simulink model "AccTarSel_PLAN_CTRL"  (R2018b)
settings: Solver=FixedStepDiscrete  StartTime=0.0  StopTime=inf  FixedStep=0.01  RelTol=1e-3
PostLoadFcn:
  | if any(exist('dsrtsu_mdlpostloadfcn', 'file') ~= 0), dsrtsu_mdlpostloadfcn('Execute', bdroot); end
undefined symbols (not defined in the file or in its folder): P_CutInEnable, P_dObjDrvOffMax, P_dObjDrvOffMin, P_dvarYMax4PO, P_dyCutInThres, P_kapHystThres, P_PlausIntegDisable, P_plausMin4PO, P_probExistMin4PO, P_StandObjEnable, P_tAxTrackNegLower, P_tAxTrackNegUpper, P_tAxTrackPosLower, P_tAxTrackPosUpper, P_tCurvFilt, P_tCutInFilt, P_tFiltAxAbsPONegFast, P_tFiltAxAbsPONegSlow, P_tFiltAxAbsPOPosFast, P_tFiltAxAbsPOPosSlow, P_tFiltAxAbsPOStand, P_tFiltVxAxPOFast, P_tFiltVxAxPOSlow, P_tMinDrvPhase, P_vObjDrvOff, P_vStandStill, P_vStandStillHyst, P_vyCutInThres
libraries: LPFilter x6, simulink x3
(part 1 of 3)
settings Model: DSRTSU_INTERNAL_RTI_VER=540  DSRTSU_INTERNAL_RTI_TYPE=rti1401  RTICANMMDATA=struct('GeneralSetupData',struct('modelroot','E:\jiangyunchengGit\laneChangeFunctional\ACC','generalsettings',struct('filesettings',struct('destfolder',struct('Name','RTICANMM_FILES','Check',1),'buildfolder',struct('Name','.','Check',1),'AbsDestfolder',struct('Name','E:\jiangyunchengGit\laneChangeFunctional\ACC\RTICANMM_FILES'),'AbsBuildfolder',struct('Name','E:\jiangyunchengGit\laneChangeFunctional\ACC'))),'options',struct('addpaths',1,'rmpaths',1,'addtrcexclusion',logical(1),'cannavigator',struct('checkmonitoring',0),'show_usrtrc',0,'use_usrtrc',0),'advanced',struct('options',ones(1,100)),'MPSetup',{{}},'RTI',struct('Type','RTI1401','Ver','7.12','Date','02-May-2019'),'modelname','AccTarSel_PLAN_CTRL','block','AccTarSel_PLAN_CTRL'))  DSRTSU_INTERNAL_RTIFPGA=130  Creator=linqi  LastModifiedBy=lenovo
settings OptimizationCC: BlockReduction=off  ConditionallyExecuteInputs=off  OptimizeBlockIOStorage=off  BufferReuse=off  GlobalBufferReuse=off  ExpressionFolding=off  PassReuseOutputArgsThreshold=0  LocalBlockOutputs=off  OptimizeDataStoreBuffers=off  BusAssignmentInplaceUpdate=off  OptimizationLevel=level0
settings DebuggingCC: ParameterTunabilityLossMsg=error
settings HardwareCC: ProdBitPerPointer=32  ProdBitPerSizeT=32  ProdBitPerPtrDiffT=32  ProdLargestAtomicInteger=Integer  ProdEndianess=BigEndian  ProdWordSize=32  ProdHWDeviceType=Custom Processor->Custom  TargetIntDivRoundTo=Zero  TargetEndianess=BigEndian  TargetHWDeviceType=Custom Processor->Custom
settings ModelReferenceCC: ModelReferenceNumInstancesAllowed=Single
settings SFSimCC: MATLABDynamicMemAlloc=off
settings RTWCC: SystemTargetFile=rti1401.tlc  MakeCommand=make_rti  TemplateMakefile=rti1401.tmf  Description=dSPACE DS1401 Hardware Platform  GenerateReport=on  LaunchReport=on
settings CodeAppCC: OperatorAnnotations=on
settings STFCustomTargetCC: ParMdlRefBuildCompliant=on  SystemTargetFile=rti1401.tlc
settings GRTTargetCC: TargetLangStandard=C89/C90 (ANSI)  CompOptLevelCompliant=off  ConcurrentExecutionCompliant=off  CombineOutputUpdateFcns=off  MatFileLogging=off  CPPClassGenCompliant=off  UseToolchainInfoCompliant=off

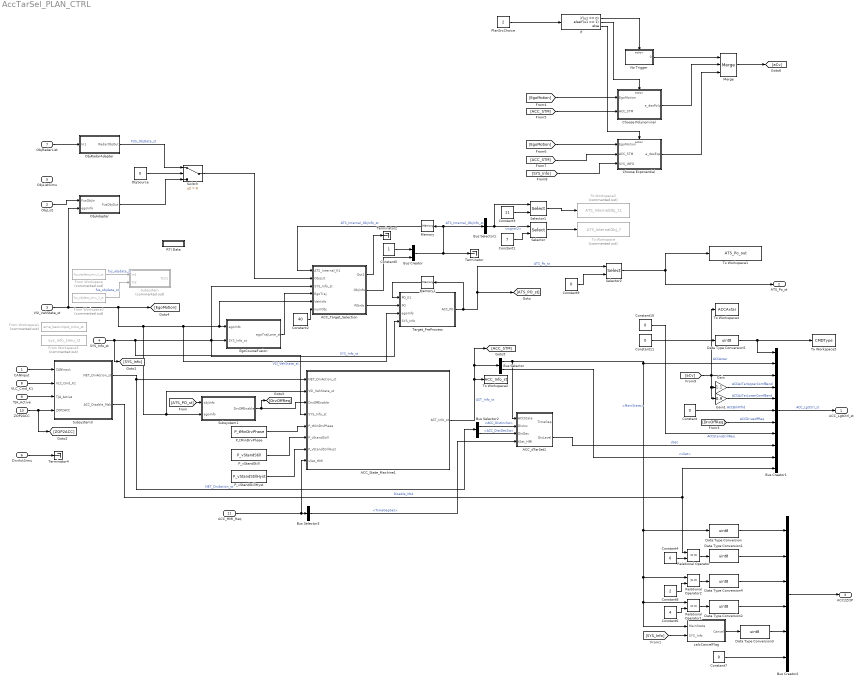
== system AccTarSel_PLAN_CTRL ==
  CANInput : Inport  OutDataTypeStr=Bus: COM_VEHBUS_ST  BusOutputAsStruct=on
  ObjList : Inport  Port=2  OutDataTypeStr=Bus: FUS_OBJ_OUTPUT_ST  BusOutputAsStruct=on
  VSI_VehState_st : Inport  Port=3  OutDataTypeStr=Bus: VSI_VEHSTATE_ST  BusOutputAsStruct=on
  SYS_Info_st : Inport  Port=4  OutDataTypeStr=Bus: SYS_INFO_ST  BusOutputAsStruct=on
  ObjListSimu : Inport  Port=5  OutDataTypeStr=Bus: FUS_OBJDATA_ST  BusOutputAsStruct=on
  DrvActSimu : Inport  Port=6  OutDataTypeStr=Bus: NET_DRVACTION_ST  BusOutputAsStruct=on
  ObjRadarList : Inport  Port=7  OutDataTypeStr=Bus: Radar410_Info_ST  BusOutputAsStruct=on
  VLC_Cmd_K1 : Inport  Port=8  OutDataTypeStr=Bus: VLC_LGTCMD_ST  BusOutputAsStruct=on
  TJA_Active : Inport  Port=9
  ZOP2ACC : Inport  Port=10  OutDataTypeStr=Bus: ZOP2ACC  BusOutputAsStruct=on
  ACC_HMI_Req : Inport  Port=11  OutDataTypeStr=Bus: ACC_HMI_REQ
  ACC_State_Machine1 : Stateflow chart  TreatAsAtomicUnit=on
  ACC_Target_Selection : Subsystem  TreatAsAtomicUnit=on
  ACC_dTarSet1 : Subsystem
  Bus Creator : BusCreator  Inputs=2  OutDataTypeStr=Bus: ATS_INTERNAL_OBJINFO_ST  NonVirtualBus=on
  Bus Creator1 : BusCreator  Inputs=11  OutDataTypeStr=Bus: ACC_LGTCTRL_ST  NonVirtualBus=on
      settings: InheritFromInputs=off
  Bus Creator2 : BusCreator  Inputs=6  OutDataTypeStr=Bus: ACC_Status_ST  NonVirtualBus=on
      settings: InheritFromInputs=off
  Bus Selector : BusSelector  OutputSignals=MainState,vSet
  Bus Selector1 : BusSelector  OutputSignals=signal2
  Bus Selector2 : BusSelector  OutputSignals=ACC_DistIncSw,ACC_DistDecSw
  Bus Selector3 : BusSelector  OutputSignals=TimeGapSet
  Choose Exponential : Subsystem  TreatAsAtomicUnit=on
  Choose Polynominal : Subsystem  TreatAsAtomicUnit=on
  Constant : Constant  Value=0  OutDataTypeStr=boolean
  Constant1 : Constant  Value=7  OutDataTypeStr=double
  Constant10 : Constant  Value=0  OutDataTypeStr=boolean
  Constant11 : Constant  Value=0  OutDataTypeStr=boolean
  Constant2 : Constant  Value=40  OutDataTypeStr=int32
  Constant3 : Constant  Value=11  OutDataTypeStr=double
  Constant4 : Constant  Value=0  OutDataTypeStr=uint16
  Constant5 : Constant  OutDataTypeStr=double
  Constant6 : Constant  Value=4  OutDataTypeStr=single
  Constant7 : Constant  Value=0  OutDataTypeStr=uint8
  Constant8 : Constant  Value=2  OutDataTypeStr=single
  Constant9 : Constant  Value=0  OutDataTypeStr=int32
  Data Type Conversion{,1..5} (6 alike) : DataTypeConversion  OutDataTypeStr=uint8
  EgoCourseFusion : Subsystem
  From Workspace : FromWorkspace  Commented=on  VariableName=fus_objdata_simu_1_st  OutDataTypeStr=Bus: FUS_OBJDATA_SIMU_ST  SampleTime=0
  From Workspace1 : FromWorkspace  Commented=on  VariableName=eme_basicinput_simu_st  OutDataTypeStr=Bus: VSI_VEHSTATE_ST  SampleTime=0
  From Workspace2 : FromWorkspace  Commented=on  VariableName=fus_objdata_simu_2_st  OutDataTypeStr=Bus: FUS_OBJDATA_SIMU_ST  SampleTime=0
  From Workspace3 : FromWorkspace  Commented=on  VariableName=sys_info_simu_st  OutDataTypeStr=Bus: SYS_INFO_ST  SampleTime=0
  Gain : Gain  Gain=1.1
  Gain1 : Gain  Gain=0.9
  If : If  IfExpression=u1 == 0  ElseIfExpressions=u1 == 1
  Memory : Memory
  Memory1 : Memory
  Merge : Merge  Inputs=3
  No Trigger : Subsystem  TreatAsAtomicUnit=on
  ObjAdapter : Subsystem
  ObjRadarAdapter : Subsystem
  ObjSource : Constant  Value=0  OutDataTypeStr=single
  P_tMinDrvPhase : Constant  Value=P_tMinDrvPhase  OutDataTypeStr=single
  P_vStandStill : Constant  Value=P_vStandStill  OutDataTypeStr=single
  P_vStandStillHyst : Constant  Value=P_vStandStillHyst  OutDataTypeStr=single
  PlanSrcChoice : Constant  Value=2
  RTI Data : Subsystem  Tag=struct('RTIDataServer',struct('RTIDataServerVs','2','RTIModelDescription','struct(''main'',''AccTarSel_PLAN_CTRL'',''sub'',''AccTarSel_PLAN_CTRL'',''isMp'',0)'))  LoadFcn="if exist('rtidc'), try,  rtidc('DataHostBlockClbLoad', gcbh); catch, disp(['Warning: ''LoadFcn'' for RTI Data block failed: ' lasterr]); end, end,"  mask(RTI_DATA_HOST){}
      mask help:
      | RTI Data Block.
      | This block is used by RTI to store internal model-dependent data.
      | Please keep this block on the root level of the model. Deleting this block will result in data loss.
      |
      | NEVER DELETE OR COPY THIS BLOCK!
      settings: CopyFcn="if exist('rtidc'), try,  rtidc('DataHostBlockClbCopy', gcbh); catch, disp(['Warning: ''CopyFcn'' for RTI Data block failed: ' lasterr]); end, end,"  DeleteFcn="if exist('rtidc'), try,  rtidc('DataHostBlockClbDelete', gcbh); catch, disp(['Warning: ''DeleteFcn'' for RTI Data block failed: ' lasterr]); end, end,"  ModelCloseFcn="if exist('rtidc'), try,  rtidc('DataHostBlockClbModelClose', gcbh); catch, disp(['Warning: ''ModelCloseFcn'' for RTI Data block failed: ' lasterr]); end, end,"  PreSaveFcn="if exist('rtidc'), try,  rtidc('DataHostBlockClbPreSave', gcbh); catch, disp(['Warning: ''PreSaveFcn'' for RTI Data block failed: ' lasterr]); end, end,"  PostSaveFcn="if exist('rtidc'), try,  rtidc('DataHostBlockClbPostSave', gcbh); catch, disp(['Warning: ''PostSaveFcn'' for RTI Data block failed: ' lasterr]); end, end,"  NameChangeFcn="if exist('rtidc'), try,  rtidc('DataHostBlockClbNameChange', gcbh); catch, disp(['Warning: ''NameChangeFcn'' for RTI Data block failed: ' lasterr]); end, end,"
      mask Help:
      | RTI Data Block.
      | This block is used by RTI to store internal model-dependent data.
      | Please keep this block on the root level of the model. Deleting this block will result in data loss.
      | 
      | NEVER DELETE OR COPY THIS BLOCK!
      mask Display:
      | text(0.5, 0.5, 'RTI Data', 'HorizontalAlignment', 'center');
      | plot([1 0]);
  Relational Operator : RelationalOperator  Operator===  OutDataTypeStr=boolean  RndMeth=Simplest
  Relational Operator1 : RelationalOperator  Operator===  OutDataTypeStr=boolean  RndMeth=Simplest
  Relational Operator2 : RelationalOperator  OutDataTypeStr=boolean  RndMeth=Simplest
  Selector : Selector  IndexMode=Zero-based  InputPortWidth=40  IndexOptions=Index vector (port)  Indices=[1 3]  OutputSizes=1
  Selector1 : Selector  IndexMode=Zero-based  InputPortWidth=40  IndexOptions=Index vector (port)  Indices=[1 3]  OutputSizes=1
  Selector2 : Selector  IndexMode=Zero-based  InputPortWidth=6  IndexOptions=Index vector (port)  Indices=[1 3]  OutputSizes=1
  Subsystem : Subsystem  Commented=on
  Subsystem1 : Subsystem
  Subsystem3 : Subsystem
  Switch : Switch  Criteria=u2 > Threshold
  Target_PreProcess : Subsystem
  Terminator : Terminator
  Terminator2 : Terminator
  Terminator4 : Terminator
  To Workspace : ToWorkspace  Commented=on  VariableName=ATS_InternalObj_7  SaveFormat=Timeseries  SampleTime=-1
  To Workspace1 : ToWorkspace  VariableName=ATS_Po_out  SaveFormat=Timeseries  SampleTime=-1
  To Workspace2 : ToWorkspace  VariableName=ACC_Info_st  SaveFormat=Timeseries  SampleTime=-1
  To Workspace3 : ToWorkspace  Commented=on  VariableName=ATS_InternalObj_11  SaveFormat=Timeseries  SampleTime=-1
  To Workspace4 : ToWorkspace  VariableName=ACCAxtar  SaveFormat=Timeseries  SampleTime=-1
  To Workspace5 : ToWorkspace  VariableName=CMDType  SaveFormat=Timeseries  SampleTime=-1
  calcCancelFlag : Subsystem
  ACC_LgtCtrl_st : Outport  OutDataTypeStr=Bus: ACC_LGTCTRL_ST  BusOutputAsStruct=on
  ATS_Po_st : Outport  Port=2  OutDataTypeStr=Bus: ATS_PO_ST  BusOutputAsStruct=on
  ACC2ZOP : Outport  Port=3  OutDataTypeStr=Bus: ACC_Status_ST  BusOutputAsStruct=on
  wires:
  EgoCourseFusion/1(egoTrajLane_st) -> ACC_Target_Selection/4(EgoTraj)
  ACC_Target_Selection/1(Out1) -> Terminator2/1
  Bus Creator/1 -> Memory/1, Bus Selector1/1, Terminator/1  "ATS_Internal_ObjInfo_st"
  Constant5/1 -> Bus Creator/1
  ACC_Target_Selection/2(ObjInfo) -> Bus Creator/2
  Target_PreProcess/1(ACC_PO) -> Memory1/1, Selector2/1, [ATS_PO_st]  "ATS_Po_st"
  ACC_State_Machine1/1(AST_Info_st) -> To Workspace2/1, [ACC_STM], Bus Selector/1  "AST_Info_st"
  VSI_VehState_st/1 -> ObjAdapter/2(egoInfo), [EgoMotion], ACC_State_Machine1/2(VSI_VehState_st), Subsystem1/2(egoInfo), Target_PreProcess/3(egoInfo), EgoCourseFusion/1(egoInfo), ACC_Target_Selection/5(VehInfo)  "VSI_VehState_st"
  [aCv] -> To Workspace4/1, Gain1/1, Gain/1, Bus Creator1/3  "ACCAxtar"
  From Workspace/1 -> Subsystem/1(In1)  "fus_objdata_st"
  From Workspace2/1 -> Subsystem/2(In2)  "fus_objdata_st"
  Constant10/1 -> Bus Creator1/8  "ACCStandstillReq"
  [ATS_PO_st] -> Subsystem1/1(objInfo)
  Subsystem1/1(DrvOffEnable) -> [DrvOffReq], ACC_State_Machine1/3(DrvOffEnable)
  P_tMinDrvPhase/1 -> ACC_State_Machine1/5(P_tMinDrvPhase)
  P_vStandStill/1 -> ACC_State_Machine1/6(P_vStandStill)
  Gain/1 -> Bus Creator1/4  "ACCAxTarUpperComfBand"
  Gain1/1 -> Bus Creator1/5  "ACCAxTarLowerComfBand"
  Constant/1 -> Bus Creator1/6  "ACCBrkPrfrd"
  [DrvOffReq] -> Bus Creator1/7  "ACCDriveoffReq"
  Bus Creator1/1 -> ACC_LgtCtrl_st/1  "ACC_LgtCtrl_st"
  SYS_Info_st/1 -> [SYS_Info], ACC_State_Machine1/4(SYS_Info_st), ACC_Target_Selection/3(SYS_Info_st), Target_PreProcess/4(SYS_Info), EgoCourseFusion/2(SYS_Info_st)  "SYS_Info_st"
  Memory/1 -> ACC_Target_Selection/1(ATS_Internal_K1)  "ATS_Internal_ObjInfo_st"
  Selector/1 -> To Workspace/1
  Constant1/1 -> Selector/2
  Bus Selector1/1 -> Selector1/1, Selector/1  "<signal2>"
  ObjList/1 -> ObjAdapter/1(FusObjIn)
  CANInput/1 -> Subsystem3/1(CANInput)
  Subsystem3/1(NET_DrvAction_st) -> ACC_State_Machine1/1(NET_DrvAction_st), Bus Selector2/1  "NET_DrvAction_st"
  DrvActSimu/1 -> Terminator4/1
  Bus Selector/2 -> Bus Creator1/10  "<vSet>"
  ObjRadarList/1 -> ObjRadarAdapter/1(In1)
  Constant2/1 -> ACC_Target_Selection/6(numObj)
  ACC_Target_Selection/3(POInfo) -> Target_PreProcess/2(PO)
  Memory1/1 -> Target_PreProcess/1(PO_K1)
  P_vStandStillHyst/1 -> ACC_State_Machine1/7(P_vStandStillHyst)
  ObjSource/1 -> Switch/2
  Switch/1 -> ACC_Target_Selection/2(ObjList)
  ObjRadarAdapter/1(RadarObjOut) -> Switch/1  "FUS_ObjData_st"
  ObjAdapter/1(FusObjOut) -> Switch/3
  VLC_Cmd_K1/1 -> Subsystem3/2(VLC_Cmd_K1)
  Selector1/1 -> To Workspace3/1
  Constant3/1 -> Selector1/2
  Bus Selector2/1 -> ACC_dTarSet1/2(DisInc)  "<ACC_DistIncSw>"
  Bus Selector2/2 -> ACC_dTarSet1/3(DisDec)  "<ACC_DistDecSw>"
  ACC_dTarSet1/2(DisLevel) -> Bus Creator1/9  "dSet"
  Subsystem3/2(ACC_Disable_Msk) -> Bus Creator1/11, Relational Operator/1  "Disable_Msk"
  TJA_Active/1 -> Subsystem3/3(TJA_Active)
  Bus Creator2/1 -> ACC2ZOP/1
  Constant4/1 -> Relational Operator/2
  Data Type Conversion/1 -> Bus Creator2/1
  Relational Operator/1 -> Data Type Conversion1/1
  Data Type Conversion1/1 -> Bus Creator2/2
  Constant6/1 -> Relational Operator1/2
  Relational Operator1/1 -> Data Type Conversion2/1
  Data Type Conversion2/1 -> Bus Creator2/4
  [SYS_Info] -> calcCancelFlag/2(SYS_Info)
  calcCancelFlag/1(Cancel) -> Data Type Conversion3/1
  Data Type Conversion3/1 -> Bus Creator2/5
  Constant7/1 -> Bus Creator2/6
  Relational Operator2/1 -> Data Type Conversion4/1
  Constant8/1 -> Relational Operator2/2
  Bus Selector/1 -> ACC_dTarSet1/1(ACCState), Bus Creator1/2, Relational Operator2/1, calcCancelFlag/1(MainState), Relational Operator1/1, Data Type Conversion/1  "<MainState>"
  Data Type Conversion4/1 -> Bus Creator2/3
  ZOP2ACC/1 -> [ZOP2ACC], Subsystem3/4(ZOP2ACC)
  Constant9/1 -> Selector2/2
  Selector2/1 -> ATS_Po_st/1, To Workspace1/1
  Bus Selector3/1 -> ACC_dTarSet1/4(tSet_HMI)  "<TimeGapSet>"
  ACC_HMI_Req/1 -> ACC_State_Machine1/8(vSet_HMI), Bus Selector3/1
  Constant11/1 -> Data Type Conversion5/1
  Data Type Conversion5/1 -> To Workspace5/1, Bus Creator1/1
  [EgoMotion] -> Choose Polynominal/1(EgoMotion)
  [ACC_STM] -> Choose Polynominal/2(ACC_STM)
  [ACC_STM] -> Choose Exponential/2(ACC_STM)
  [EgoMotion] -> Choose Exponential/1(EgoMotion)
  [SYS_Info] -> Choose Exponential/3(SYS_INFO)
  Merge/1 -> [aCv]
  PlanSrcChoice/1 -> If/1
  If/1 -> No Trigger/Action
  If/2 -> Choose Polynominal/Action
  If/3 -> Choose Exponential/Action
  No Trigger/1(0) -> Merge/1
  Choose Polynominal/1(a_desPoly) -> Merge/2
  Choose Exponential/1(a_desExp) -> Merge/3

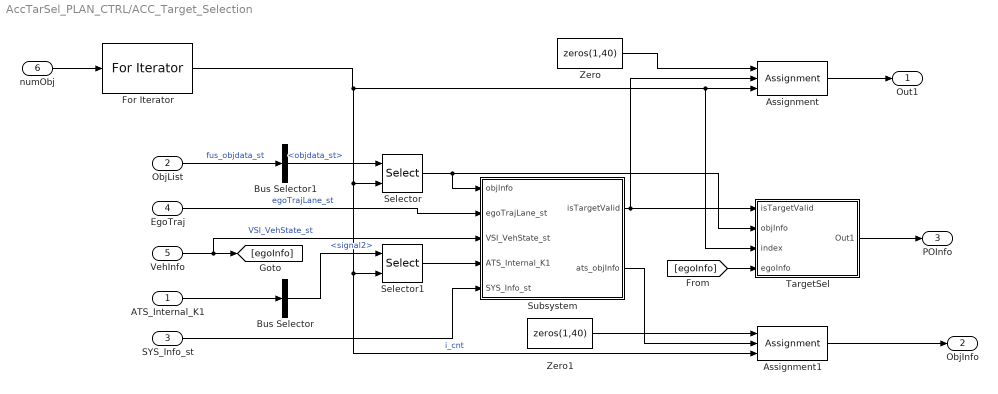
== system AccTarSel_PLAN_CTRL/ACC_Target_Selection ==
  ATS_Internal_K1 : Inport
  ObjList : Inport  Port=2
  SYS_Info_st : Inport  Port=3
  EgoTraj : Inport  Port=4
  VehInfo : Inport  Port=5
  numObj : Inport  Port=6
  Assignment : Assignment  IndexMode=Zero-based  DiagnosticForDimensions=Warning  IndexOptions=Index vector (port)  Indices=1  OutputSizes=1
  Assignment1 : Assignment  IndexMode=Zero-based  DiagnosticForDimensions=Warning  IndexOptions=Index vector (port)  Indices=1  OutputSizes=1
  Bus Selector : BusSelector  OutputSignals=signal2
  Bus Selector1 : BusSelector  OutputSignals=objdata_st
  For Iterator : ForIterator  IterationSource=external  IterationLimit=2  IndexMode=Zero-based
  Selector : Selector  IndexMode=Zero-based  InputPortWidth=40  IndexOptions=Index vector (port)  Indices=[1 3]  OutputSizes=1
  Selector1 : Selector  IndexMode=Zero-based  InputPortWidth=40  IndexOptions=Index vector (port)  Indices=[1 3]  OutputSizes=1
  Subsystem : Subsystem
  TargetSel : Subsystem
  Zero : Constant  Value=zeros(1,40)  OutDataTypeStr=boolean
  Zero1 : Constant  Value=zeros(1,40)  OutDataTypeStr=Bus: ATS_OBJINFO_ST
  Out1 : Outport
  ObjInfo : Outport  Port=2  OutDataTypeStr=Bus: ATS_OBJINFO_ST
  POInfo : Outport  Port=3  OutDataTypeStr=Bus: ATS_PO_ST
  wires:
  For Iterator/1 -> Selector1/2, Assignment1/3, Selector/2, Assignment/3, TargetSel/3(index)  "i_cnt"
  ObjList/1 -> Bus Selector1/1  "fus_objdata_st"
  Bus Selector1/1 -> Selector/1  "<objdata_st>"
  Selector/1 -> Subsystem/1(objInfo), TargetSel/2(objInfo)
  Zero/1 -> Assignment/1
  Assignment/1 -> Out1/1
  Zero1/1 -> Assignment1/1
  Assignment1/1 -> ObjInfo/1
  Subsystem/1(isTargetValid) -> Assignment/2, TargetSel/1(isTargetValid)
  EgoTraj/1 -> Subsystem/2(egoTrajLane_st)  "egoTrajLane_st"
  VehInfo/1 -> [egoInfo], Subsystem/3(VSI_VehState_st)  "VSI_VehState_st"
  Subsystem/2("ats_objInfo ") -> Assignment1/2
  Selector1/1 -> Subsystem/4(ATS_Internal_K1)
  ATS_Internal_K1/1 -> Bus Selector/1
  Bus Selector/1 -> Selector1/1  "<signal2>"
  SYS_Info_st/1 -> Subsystem/5(SYS_Info_st)
  numObj/1 -> For Iterator/1
  TargetSel/1(Out1) -> POInfo/1
  [egoInfo] -> TargetSel/4(egoInfo)

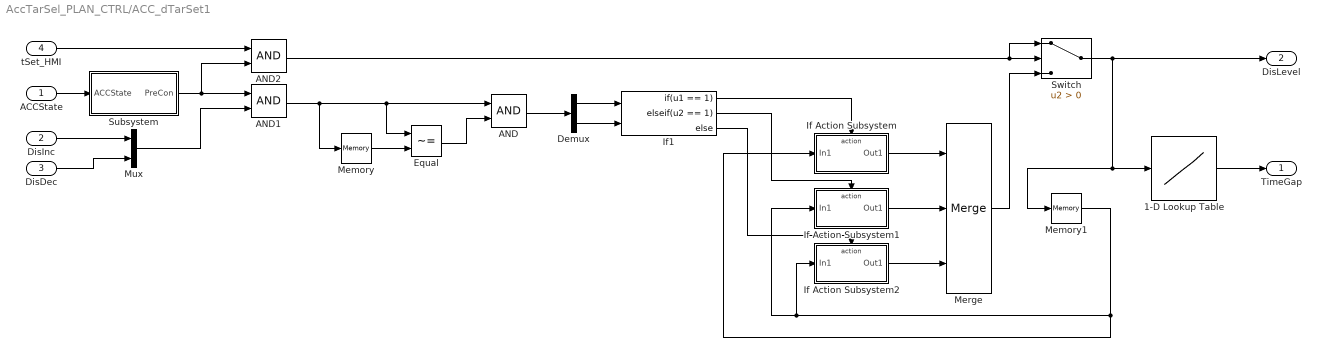
== system AccTarSel_PLAN_CTRL/ACC_dTarSet1 ==
  ACCState : Inport
  DisInc : Inport  Port=2
  DisDec : Inport  Port=3
  tSet_HMI : Inport  Port=4
  1-D Lookup Table : Lookup_n-D  NumberOfTableDimensions=1  BreakpointsForDimension1=[1 2 3]  Table=[1.2 1.8 2.1]  InterpMethod=Flat  InternalRulePriority=Speed  RndMeth=Simplest  InputSameDT=on
  AND : Logic  AllPortsSameDT=off  OutDataTypeStr=boolean
  AND1 : Logic  AllPortsSameDT=off  OutDataTypeStr=boolean
  AND2 : Logic  AllPortsSameDT=off  OutDataTypeStr=boolean
  Demux : Demux  Outputs=2
  Equal : RelationalOperator  Operator=~=  OutDataTypeStr=boolean  RndMeth=Simplest
  If Action Subsystem : Subsystem  TreatAsAtomicUnit=on
  If Action Subsystem1 : Subsystem  TreatAsAtomicUnit=on
  If Action Subsystem2 : Subsystem  TreatAsAtomicUnit=on
  If1 : If  NumInputs=2  IfExpression=u1 == 1  ElseIfExpressions=u2 == 1
  Memory : Memory
  Memory1 : Memory  InitialCondition=3
  Merge : Merge  Inputs=3  InitialOutput=0
  Mux : Mux  Inputs=2
  Subsystem : Subsystem
  Switch : Switch  Criteria=u2 > Threshold
  TimeGap : Outport
  DisLevel : Outport  Port=2
  wires:
  If1/1 -> If Action Subsystem/Action
  If Action Subsystem/1(Out1) -> Merge/1
  Memory1/1 -> If Action Subsystem/1(In1), If Action Subsystem1/1(In1), If Action Subsystem2/1(In1)
  If Action Subsystem1/1(Out1) -> Merge/2
  If1/2 -> If Action Subsystem1/Action
  If Action Subsystem2/1(Out1) -> Merge/3
  If1/3 -> If Action Subsystem2/Action
  Subsystem/1(PreCon) -> AND2/2, AND1/1
  AND1/1 -> Memory/1, Equal/1, AND/1
  Memory/1 -> Equal/2
  Equal/1 -> AND/2
  AND/1 -> Demux/1
  Demux/1 -> If1/1
  Demux/2 -> If1/2
  Mux/1 -> AND1/2
  ACCState/1 -> Subsystem/1(ACCState)
  DisInc/1 -> Mux/1
  DisDec/1 -> Mux/2
  1-D Lookup Table/1 -> TimeGap/1
  Switch/1 -> DisLevel/1, Memory1/1, 1-D Lookup Table/1
  Merge/1 -> Switch/3
  tSet_HMI/1 -> AND2/1
  AND2/1 -> Switch/1, Switch/2

== system AccTarSel_PLAN_CTRL/Choose Exponential ==
  EgoMotion : Inport
  ACC_STM : Inport  Port=2
  SYS_INFO : Inport  Port=3
  Action Port : ActionPort  ActionType=else
  Exponential : Subsystem
  a_desExp : Outport
  wires:
  ACC_STM/1 -> Exponential/2(ACC_STM)
  EgoMotion/1 -> Exponential/1(EgoMotion)
  Exponential/1(aCmd) -> a_desExp/1
  SYS_INFO/1 -> Exponential/3(SYS_Info)

== system AccTarSel_PLAN_CTRL/Choose Polynominal ==
  EgoMotion : Inport
  ACC_STM : Inport  Port=2
  Action Port : ActionPort  ActionType=elseif
  Polynominal : Subsystem
  a_desPoly : Outport
  wires:
  Polynominal/1(a_des) -> a_desPoly/1
  EgoMotion/1 -> Polynominal/1(EgoMotion)
  ACC_STM/1 -> Polynominal/2(ACC_STM)

== system AccTarSel_PLAN_CTRL/EgoCourseFusion ==
  egoInfo : Inport
  SYS_Info_st : Inport  Port=2
  Bus Creator : BusCreator  Inputs=4  OutDataTypeStr=Bus: TRAJ_LANE_ST
  Bus Selector : BusSelector  OutputSignals=Curvature
  Bus Selector1 : BusSelector  OutputSignals=dT
  Constant2 : Constant  Value=0.5  OutDataTypeStr=single
  Constant3 : Constant  Value=0  OutDataTypeStr=single
  Constant4 : Constant  Value=0  OutDataTypeStr=single
  Constant5 : Constant  Value=0  OutDataTypeStr=single
  CurvatureFilt : Subsystem
  Multiply : Product
  egoTrajLane_st : Outport
  wires:
  Bus Creator/1 -> egoTrajLane_st/1  "egoTrajLane_st"
  CurvatureFilt/1(kapTrajFilt) -> Multiply/1  "kapTrajFilt"
  Constant2/1 -> Multiply/2
  Constant4/1 -> Bus Creator/3  "c"
  Constant3/1 -> Bus Creator/1  "a"
  Multiply/1 -> Bus Creator/2  "b"
  Constant5/1 -> Bus Creator/4  "d"
  egoInfo/1 -> Bus Selector/1
  Bus Selector/1 -> CurvatureFilt/1(In1)  "<Curvature>"
  SYS_Info_st/1 -> Bus Selector1/1
  Bus Selector1/1 -> CurvatureFilt/2(In2)  "<dT>"

== system AccTarSel_PLAN_CTRL/No Trigger ==
  Action Port : ActionPort  ActionType=then
  Constant : Constant  Value=0  OutDataTypeStr=single
  0 : Outport
  wires:
  Constant/1 -> 0/1

== system AccTarSel_PLAN_CTRL/ObjAdapter ==
  FusObjIn : Inport
  egoInfo : Inport  Port=2
  Bus Creator : BusCreator  Inputs=2  OutDataTypeStr=Bus: FUS_OBJDATA_ST  NonVirtualBus=on
  Bus Selector : BusSelector  OutputSignals=objects
  Constant : Constant  Value=0  OutDataTypeStr=double
  For Each Subsystem : Subsystem  TreatAsAtomicUnit=on
  FusObjOut : Outport  OutDataTypeStr=Bus: FUS_OBJDATA_ST
  wires:
  FusObjIn/1 -> Bus Selector/1
  Bus Selector/1 -> For Each Subsystem/1(In1)  "<objects>"
  Bus Creator/1 -> FusObjOut/1
  For Each Subsystem/1(Out1) -> Bus Creator/2  "objdata_st"
  Constant/1 -> Bus Creator/1  "timeStamp"
  egoInfo/1 -> For Each Subsystem/2(In2)

== system AccTarSel_PLAN_CTRL/ObjRadarAdapter ==
  In1 : Inport
  Bus Creator : BusCreator  Inputs=2  OutDataTypeStr=Bus: FUS_OBJDATA_ST  NonVirtualBus=on
      settings: InheritFromInputs=off
  Bus Selector : BusSelector  OutputSignals=x50_20_Obj_00,x51_21_Obj_01,x52_22_Obj_02,x53_23_Obj_03,x54_24_Obj_04,x55_25_Obj_05,x56_26_Obj_06,x57_27_Obj_07,x58_28_Obj_08,x59_29_Obj_09,x5A_2A_Obj_10,x5B_2B_Obj_11,x5C_2C_Obj_12,x5D_2D_Obj_13,x5E_2E_Obj_14,x5F_2F_Obj_15,x60_30_Obj_16,x61_31_Obj_17,x62_32_Obj_18,x63_33_Obj_19,x64_34_Obj_20,x65_35_Obj_21,x66_36_Obj_22,x67_37_Obj_23,x68_38_Obj_24,x69_39_Obj_25,x6A_3A_Obj_26,x6B_3B_Obj_27,x6C_3C_Obj_28,x6D_3D_Obj_29,x6E_3E_Obj_30,x6F_3F_Obj_31,x70_40_Obj_32,x71_41_Obj_33,x72_42_Obj_34,x73_43_Obj_35,x74_44_Obj_36,x75_45_Obj_37,x76_46_Obj_38,x77_47_Obj_39
  Constant : Constant  Value=0  OutDataTypeStr=double
  For Each Subsystem : Subsystem  TreatAsAtomicUnit=on
  Vector Concatenate : Concatenate  NumInputs=40
  RadarObjOut : Outport  OutDataTypeStr=Bus: FUS_OBJDATA_ST
  wires:
  In1/1 -> Bus Selector/1
  Bus Selector/1 -> Vector Concatenate/1  "<x50_20_Obj_00>"
  Bus Selector/2 -> Vector Concatenate/2  "<x51_21_Obj_01>"
  Bus Selector/3 -> Vector Concatenate/3  "<x52_22_Obj_02>"
  Bus Selector/4 -> Vector Concatenate/4  "<x53_23_Obj_03>"
  Bus Selector/5 -> Vector Concatenate/5  "<x54_24_Obj_04>"
  Bus Selector/6 -> Vector Concatenate/6  "<x55_25_Obj_05>"
  Bus Selector/7 -> Vector Concatenate/7  "<x56_26_Obj_06>"
  Bus Selector/8 -> Vector Concatenate/8  "<x57_27_Obj_07>"
  Bus Selector/9 -> Vector Concatenate/9  "<x58_28_Obj_08>"
  Bus Selector/10 -> Vector Concatenate/10  "<x59_29_Obj_09>"
  Bus Selector/11 -> Vector Concatenate/11  "<x5A_2A_Obj_10>"
  Bus Selector/12 -> Vector Concatenate/12  "<x5B_2B_Obj_11>"
  Bus Selector/13 -> Vector Concatenate/13  "<x5C_2C_Obj_12>"
  Bus Selector/14 -> Vector Concatenate/14  "<x5D_2D_Obj_13>"
  Bus Selector/15 -> Vector Concatenate/15  "<x5E_2E_Obj_14>"
  Bus Selector/16 -> Vector Concatenate/16  "<x5F_2F_Obj_15>"
  Bus Selector/17 -> Vector Concatenate/17  "<x60_30_Obj_16>"
  Bus Selector/18 -> Vector Concatenate/18  "<x61_31_Obj_17>"
  Bus Selector/19 -> Vector Concatenate/19  "<x62_32_Obj_18>"
  Bus Selector/20 -> Vector Concatenate/20  "<x63_33_Obj_19>"
  Bus Selector/21 -> Vector Concatenate/21  "<x64_34_Obj_20>"
  Bus Selector/22 -> Vector Concatenate/22  "<x65_35_Obj_21>"
  Bus Selector/23 -> Vector Concatenate/23  "<x66_36_Obj_22>"
  Bus Selector/24 -> Vector Concatenate/24  "<x67_37_Obj_23>"
  Bus Selector/25 -> Vector Concatenate/25  "<x68_38_Obj_24>"
  Bus Selector/26 -> Vector Concatenate/26  "<x69_39_Obj_25>"
  Bus Selector/27 -> Vector Concatenate/27  "<x6A_3A_Obj_26>"
  Bus Selector/28 -> Vector Concatenate/28  "<x6B_3B_Obj_27>"
  Bus Selector/29 -> Vector Concatenate/29  "<x6C_3C_Obj_28>"
  Bus Selector/30 -> Vector Concatenate/30  "<x6D_3D_Obj_29>"
  Bus Selector/31 -> Vector Concatenate/31  "<x6E_3E_Obj_30>"
  Bus Selector/32 -> Vector Concatenate/32  "<x6F_3F_Obj_31>"
  Bus Selector/33 -> Vector Concatenate/33  "<x70_40_Obj_32>"
  Bus Selector/34 -> Vector Concatenate/34  "<x71_41_Obj_33>"
  Bus Selector/35 -> Vector Concatenate/35  "<x72_42_Obj_34>"
  Bus Selector/36 -> Vector Concatenate/36  "<x73_43_Obj_35>"
  Bus Selector/37 -> Vector Concatenate/37  "<x74_44_Obj_36>"
  Bus Selector/38 -> Vector Concatenate/38  "<x75_45_Obj_37>"
  Bus Selector/39 -> Vector Concatenate/39  "<x76_46_Obj_38>"
  Bus Selector/40 -> Vector Concatenate/40  "<x77_47_Obj_39>"
  Vector Concatenate/1 -> For Each Subsystem/1(In1)
  For Each Subsystem/1(Out1) -> Bus Creator/2  "objdata_st"
  Bus Creator/1 -> RadarObjOut/1
  Constant/1 -> Bus Creator/1  "timeStamp"

== system AccTarSel_PLAN_CTRL/RTI Data ==
  RTI Data Store : Subsystem  Tag=struct('private',struct('version',struct('dsVer',uint32(2)),'access',struct('modified',['03-Feb-2021 15:51:46'],'type','Model','isPerm',1)),'public',struct('main',struct('data',[]),'sub',struct('name','','data',[])))  mask(RTI_DATA_STORE){}
      mask help:
      | RTI Data Store Block. This block is used by RTI to store internal model dependent data. Deleting this block will result in data loss.
      |
      | NEVER DELETE, COPY, OR MODIFY THIS BLOCK!
      mask Help:
      | RTI Data Store Block. This block is used by RTI to store internal model dependent data. Deleting this block will result in data loss.
      | 
      | NEVER DELETE, COPY, OR MODIFY THIS BLOCK!
      mask Display: text(0.5, 0.5, ' ', 'HorizontalAlignment', 'center');

== system AccTarSel_PLAN_CTRL/Subsystem ==
  In1 : Inport
  In2 : Inport  Port=2
  Bus Creator : BusCreator  Inputs=2  OutDataTypeStr=Bus: FUS_OBJDATA_ST  NonVirtualBus=on
  Bus Selector : BusSelector  OutputSignals=timeStamp,objdata_st
  Bus Selector1 : BusSelector  OutputSignals=objdata_st
  Vector Concatenate : Concatenate  ConcatenateDimension=2
  Out1 : Outport
  wires:
  In1/1 -> Bus Selector/1
  In2/1 -> Bus Selector1/1
  Bus Selector1/1 -> Vector Concatenate/2  "<objdata_st>"
  Bus Selector/2 -> Vector Concatenate/1  "<objdata_st>"
  Bus Selector/1 -> Bus Creator/1  "<timeStamp>"
  Vector Concatenate/1 -> Bus Creator/2  "objdata_st"
  Bus Creator/1 -> Out1/1

== system AccTarSel_PLAN_CTRL/Subsystem1 ==
  objInfo : Inport
  egoInfo : Inport  Port=2
  AND2 : Logic  AllPortsSameDT=off  OutDataTypeStr=boolean
  AND3 : Logic  Operator=OR  AllPortsSameDT=off  OutDataTypeStr=boolean
  Add : Sum
  Bus Selector : BusSelector  OutputSignals=Valid,dx,vx
  Bus Selector1 : BusSelector  OutputSignals=vRef
  Constant : Constant  OutDataTypeStr=boolean
  Constant1 : Constant  Value=0  OutDataTypeStr=int32
  If : If  IfExpression=u1 == 1
  If Action Subsystem : Subsystem  TreatAsAtomicUnit=on
  If Action Subsystem1 : Subsystem  TreatAsAtomicUnit=on
  Merge : Merge
  P_dObjDrvOffMax : Constant  Value=P_dObjDrvOffMax
  P_dObjDrvOffMin : Constant  Value=P_dObjDrvOffMin
  P_vObjDrvOff : Constant  Value=P_vObjDrvOff
  Relational Operator6 : RelationalOperator  Operator=>  OutDataTypeStr=boolean  RndMeth=Simplest
  Relational Operator7 : RelationalOperator  Operator=>  OutDataTypeStr=boolean  RndMeth=Simplest
  Relational Operator8 : RelationalOperator  Operator=>  OutDataTypeStr=boolean  RndMeth=Simplest
  Selector1 : Selector  IndexMode=Zero-based  InputPortWidth=6  IndexOptions=Index vector (port)  Indices=[1 3]  OutputSizes=1
  DrvOffEnable : Outport
  wires:
  AND2/1 -> AND3/2
  Relational Operator8/1 -> AND2/2
  Add/1 -> Relational Operator8/1  "vAbsObj"
  P_dObjDrvOffMin/1 -> Relational Operator7/2
  Relational Operator7/1 -> AND2/1
  Relational Operator6/1 -> AND3/1
  P_vObjDrvOff/1 -> Relational Operator8/2
  P_dObjDrvOffMax/1 -> Relational Operator6/2
  Bus Selector/1 -> If/1  "<Valid>"
  egoInfo/1 -> Bus Selector1/1
  Bus Selector1/1 -> Add/2  "<vRef>"
  Bus Selector/3 -> Add/1  "<vx>"
  Bus Selector/2 -> Relational Operator6/1, Relational Operator7/1  "<dx>"
  AND3/1 -> If Action Subsystem/1(In1)
  Constant/1 -> If Action Subsystem1/1(In1)
  If/1 -> If Action Subsystem/Action
  If/2 -> If Action Subsystem1/Action
  If Action Subsystem/1(Out1) -> Merge/1
  If Action Subsystem1/1(Out1) -> Merge/2
  Merge/1 -> DrvOffEnable/1  "DrvOffEnable"
  objInfo/1 -> Selector1/1
  Constant1/1 -> Selector1/2
  Selector1/1 -> Bus Selector/1

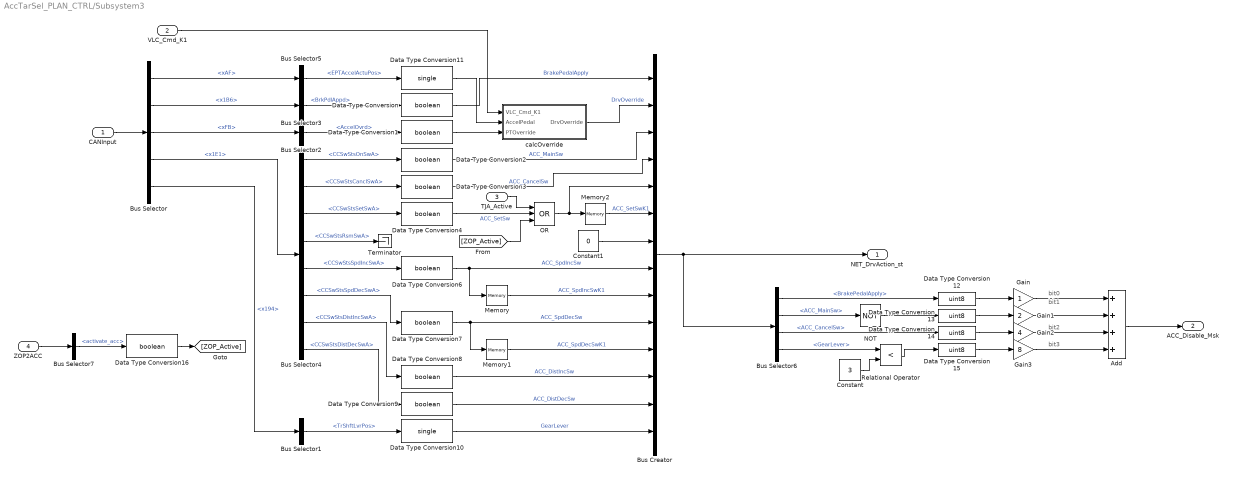
== system AccTarSel_PLAN_CTRL/Subsystem3 ==
  note: bit0
  note: bit1
  note: bit2
  note: bit3
  CANInput : Inport
  VLC_Cmd_K1 : Inport  Port=2
  TJA_Active : Inport  Port=3
  ZOP2ACC : Inport  Port=4
  Add : Sum  Inputs=++++  AccumDataTypeStr=uint16
  Bus Creator : BusCreator  Inputs=14  OutDataTypeStr=Bus: NET_DRVACTION_ST  NonVirtualBus=on
      settings: InheritFromInputs=off
  Bus Selector : BusSelector  OutputSignals=xAF,x1B6,xFB,x1E1,x194
  Bus Selector1 : BusSelector  OutputSignals=TrShftLvrPos
  Bus Selector2 : BusSelector  OutputSignals=AccelOvrd
  Bus Selector3 : BusSelector  OutputSignals=BrkPdlAppd
  Bus Selector4 : BusSelector  OutputSignals=CCSwStsOnSwA,CCSwStsCanclSwA,CCSwStsSetSwA,CCSwStsRsmSwA,CCSwStsSpdIncSwA,CCSwStsSpdDecSwA,CCSwStsDistIncSwA,CCSwStsDistDecSwA
  Bus Selector5 : BusSelector  OutputSignals=EPTAccelActuPos
  Bus Selector6 : BusSelector  OutputSignals=BrakePedalApply,ACC_MainSw,ACC_CancelSw,GearLever
  Bus Selector7 : BusSelector  OutputSignals=activate_acc
  Constant : Constant  Value=3  OutDataTypeStr=single
  Constant1 : Constant  Value=0  OutDataTypeStr=boolean
  Data Type Conversion{,1..4,6..9,16} (10 alike) : DataTypeConversion  OutDataTypeStr=boolean
  Data Type Conversion10 : DataTypeConversion  OutDataTypeStr=single
  Data Type Conversion11 : DataTypeConversion  OutDataTypeStr=single
  Data Type Conversion{12..15} (4 alike) : DataTypeConversion  OutDataTypeStr=uint8
  Gain : Gain  OutDataTypeStr=uint16
  Gain1 : Gain  Gain=2  OutDataTypeStr=uint16
  Gain2 : Gain  Gain=4  OutDataTypeStr=uint16
  Gain3 : Gain  Gain=8  OutDataTypeStr=uint16
  Memory : Memory
  Memory1 : Memory
  Memory2 : Memory
  NOT : Logic  Operator=NOT  AllPortsSameDT=off  OutDataTypeStr=boolean
  OR : Logic  Operator=OR  Inputs=3  AllPortsSameDT=off  OutDataTypeStr=boolean
  Relational Operator : RelationalOperator  Operator=<  OutDataTypeStr=boolean  RndMeth=Simplest
  Terminator : Terminator
  calcOverride : Subsystem
  NET_DrvAction_st : Outport  OutDataTypeStr=Bus: NET_DRVACTION_ST
  ACC_Disable_Msk : Outport  Port=2
  wires:
  CANInput/1 -> Bus Selector/1
  Bus Selector/5 -> Bus Selector1/1  "<x194>"
  Bus Selector/3 -> Bus Selector2/1  "<xFB>"
  Bus Selector/2 -> Bus Selector3/1  "<x1B6>"
  Bus Selector/4 -> Bus Selector4/1  "<x1E1>"
  Bus Selector3/1 -> Data Type Conversion/1  "<BrkPdlAppd>"
  Data Type Conversion/1 -> Bus Creator/1  "BrakePedalApply"
  Bus Selector2/1 -> Data Type Conversion1/1  "<AccelOvrd>"
  Bus Selector4/1 -> Data Type Conversion2/1  "<CCSwStsOnSwA>"
  Bus Selector4/2 -> Data Type Conversion3/1  "<CCSwStsCanclSwA>"
  Bus Selector4/3 -> Data Type Conversion4/1  "<CCSwStsSetSwA>"
  Bus Selector4/4 -> Terminator/1  "<CCSwStsRsmSwA>"
  Bus Selector4/5 -> Data Type Conversion6/1  "<CCSwStsSpdIncSwA>"
  Bus Selector4/6 -> Data Type Conversion7/1  "<CCSwStsSpdDecSwA>"
  Data Type Conversion6/1 -> Bus Creator/8, Memory/1  "ACC_SpdIncSw"
  Memory/1 -> Bus Creator/9  "ACC_SpdIncSwK1"
  Data Type Conversion7/1 -> Memory1/1, Bus Creator/10  "ACC_SpdDecSw"
  Memory1/1 -> Bus Creator/11  "ACC_SpdDecSwK1"
  Data Type Conversion8/1 -> Bus Creator/12  "ACC_DistIncSw"
  Bus Selector4/7 -> Data Type Conversion8/1  "<CCSwStsDistIncSwA>"
  Data Type Conversion9/1 -> Bus Creator/13  "ACC_DistDecSw"
  Bus Selector4/8 -> Data Type Conversion9/1  "<CCSwStsDistDecSwA>"
  Data Type Conversion2/1 -> Bus Creator/3  "ACC_MainSw"
  Data Type Conversion3/1 -> Bus Creator/4  "ACC_CancelSw"
  Bus Creator/1 -> Bus Selector6/1, NET_DrvAction_st/1
  Data Type Conversion10/1 -> Bus Creator/14  "GearLever"
  Bus Selector1/1 -> Data Type Conversion10/1  "<TrShftLvrPos>"
  Bus Selector/1 -> Bus Selector5/1  "<xAF>"
  Bus Selector5/1 -> Data Type Conversion11/1  "<EPTAccelActuPos>"
  calcOverride/1(DrvOverride) -> Bus Creator/2  "DrvOverride"
  VLC_Cmd_K1/1 -> calcOverride/1(VLC_Cmd_K1)
  Data Type Conversion11/1 -> calcOverride/2(AccelPedal)
  Data Type Conversion1/1 -> calcOverride/3(PTOverride)
  Memory2/1 -> Bus Creator/6  "ACC_SetSwK1"
  Bus Selector6/1 -> Data Type Conversion12/1  "<BrakePedalApply>"
  Bus Selector6/3 -> Data Type Conversion14/1  "<ACC_CancelSw>"
  Bus Selector6/2 -> NOT/1  "<ACC_MainSw>"
  NOT/1 -> Data Type Conversion13/1
  Bus Selector6/4 -> Relational Operator/1  "<GearLever>"
  Constant/1 -> Relational Operator/2
  Relational Operator/1 -> Data Type Conversion15/1
  Data Type Conversion12/1 -> Gain/1
  Data Type Conversion13/1 -> Gain1/1
  Data Type Conversion14/1 -> Gain2/1
  Data Type Conversion15/1 -> Gain3/1
  Gain/1 -> Add/1
  Gain1/1 -> Add/2
  Gain2/1 -> Add/3
  Gain3/1 -> Add/4
  Add/1 -> ACC_Disable_Msk/1
  TJA_Active/1 -> OR/1
  Data Type Conversion4/1 -> OR/2  "ACC_SetSw"
  OR/1 -> Bus Creator/5, Memory2/1
  Constant1/1 -> Bus Creator/7
  ZOP2ACC/1 -> Bus Selector7/1
  Bus Selector7/1 -> Data Type Conversion16/1  "<activate_acc>"
  Data Type Conversion16/1 -> [ZOP_Active]
  [ZOP_Active] -> OR/3

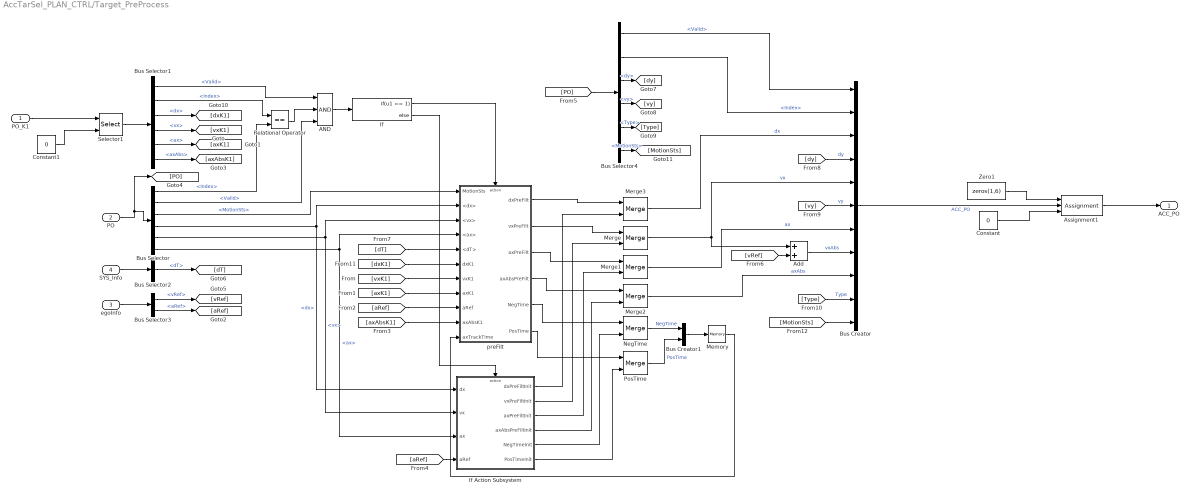
== system AccTarSel_PLAN_CTRL/Target_PreProcess ==
  PO_K1 : Inport
  PO : Inport  Port=2
  egoInfo : Inport  Port=3
  SYS_Info : Inport  Port=4
  AND : Logic  Inputs=3  AllPortsSameDT=off  OutDataTypeStr=boolean
  Add : Sum
  Assignment1 : Assignment  IndexMode=Zero-based  DiagnosticForDimensions=Warning  IndexOptions=Index vector (port)  Indices=1  OutputSizes=1
  Bus Creator : BusCreator  Inputs=11  OutDataTypeStr=Bus: ATS_PO_ST  NonVirtualBus=on
      settings: InheritFromInputs=off
  Bus Creator1 : BusCreator  Inputs=2
  Bus Selector : BusSelector  OutputSignals=Index,Valid,MotionSts,dx,vx,ax
  Bus Selector1 : BusSelector  OutputSignals=Valid,Index,dx,vx,ax,axAbs
  Bus Selector2 : BusSelector  OutputSignals=dT
  Bus Selector3 : BusSelector  OutputSignals=vRef,aRef
  Bus Selector4 : BusSelector  OutputSignals=Valid,Index,dy,vy,Type,MotionSts
  Constant : Constant  Value=0  OutDataTypeStr=int32
  Constant1 : Constant  Value=0  OutDataTypeStr=int32
  If : If  IfExpression=u1 == 1
  If Action Subsystem : Subsystem  TreatAsAtomicUnit=on
  Memory : Memory
  Merge{,1..3} (4 alike) : Merge
  NegTime : Merge
  PosTime : Merge
  Relational Operator : RelationalOperator  Operator===  OutDataTypeStr=boolean  RndMeth=Simplest
  Selector1 : Selector  IndexMode=Zero-based  InputPortWidth=6  IndexOptions=Index vector (port)  Indices=[1 3]  OutputSizes=1
  Zero1 : Constant  Value=zeros(1,6)  OutDataTypeStr=Bus: ATS_PO_ST
  preFilt : Subsystem
  ACC_PO : Outport  OutDataTypeStr=Bus: ATS_PO_ST
  wires:
  PO/1 -> [PO], Bus Selector/1
  Bus Selector1/1 -> AND/1  "<Valid>"
  Bus Selector1/2 -> Relational Operator/1  "<Index>"
  Bus Selector/1 -> Relational Operator/2  "<Index>"
  Relational Operator/1 -> AND/2
  Bus Selector/2 -> AND/3  "<Valid>"
  SYS_Info/1 -> Bus Selector2/1
  Bus Selector1/4 -> [vxK1]  "<vx>"
  Bus Selector1/5 -> [axK1]  "<ax>"
  AND/1 -> If/1
  Bus Selector/5 -> preFilt/3(<vx>), If Action Subsystem/2(vx)  "<vx>"
  Bus Selector/6 -> preFilt/4(<ax>), If Action Subsystem/3(ax)  "<ax>"
  [vxK1] -> preFilt/7(vxK1)
  [axK1] -> preFilt/8(axK1)
  If/1 -> preFilt/Action
  If/2 -> If Action Subsystem/Action
  preFilt/2(vxPreFilt) -> Merge/1
  If Action Subsystem/2(vxPreFiltInit) -> Merge/2
  preFilt/3(axPreFilt) -> Merge1/1
  If Action Subsystem/3(axPreFiltInit) -> Merge1/2
  egoInfo/1 -> Bus Selector3/1
  Bus Selector3/2 -> [aRef]  "<aRef>"
  [aRef] -> preFilt/9(aRef)
  Bus Selector1/6 -> [axAbsK1]  "<axAbs>"
  [axAbsK1] -> preFilt/10(axAbsK1)
  [aRef] -> If Action Subsystem/4(aRef)
  preFilt/4(axAbsPreFilt) -> Merge2/1
  If Action Subsystem/4(axAbsPreFiltInit) -> Merge2/2
  [PO] -> Bus Selector4/1
  Bus Selector4/1 -> Bus Creator/1  "<Valid>"
  Bus Selector4/2 -> Bus Creator/2  "<Index>"
  Merge/1 -> Bus Creator/5, Add/1  "vx"
  Merge1/1 -> Bus Creator/7  "ax"
  Merge2/1 -> Bus Creator/9  "axAbs"
  Bus Creator/1 -> Assignment1/2  "ACC_PO"
  Bus Selector3/1 -> [vRef]  "<vRef>"
  Add/1 -> Bus Creator/8  "vxAbs"
  [vRef] -> Add/2
  Bus Selector/4 -> preFilt/2(<dx>), If Action Subsystem/1(dx)  "<dx>"
  [dxK1] -> preFilt/6(dxK1)
  Bus Selector2/1 -> [dT]  "<dT>"
  [dT] -> preFilt/5(<dT>)
  preFilt/1(dxPreFilt) -> Merge3/1
  If Action Subsystem/1(dxPreFiltInit) -> Merge3/2
  Merge3/1 -> Bus Creator/3  "dx"
  Bus Selector4/3 -> [dy]  "<dy>"
  [dy] -> Bus Creator/4  "dy"
  Bus Selector4/4 -> [vy]  "<vy>"
  [vy] -> Bus Creator/6  "vy"
  Bus Selector4/5 -> [Type]  "<Type>"
  [Type] -> Bus Creator/10  "Type"
  Bus Selector1/3 -> [dxK1]  "<dx>"
  Bus Selector4/6 -> [MotionSts]  "<MotionSts>"
  [MotionSts] -> Bus Creator/11
  preFilt/5(NegTime) -> NegTime/1
  If Action Subsystem/5(NegTimeInit) -> NegTime/2
  preFilt/6(PosTime) -> PosTime/1
  If Action Subsystem/6(PosTimeInit) -> PosTime/2
  NegTime/1 -> Bus Creator1/1  "NegTime"
  PosTime/1 -> Bus Creator1/2  "PosTime"
  Bus Creator1/1 -> Memory/1
  Memory/1 -> preFilt/11(axTrackTime)
  Bus Selector/3 -> preFilt/1(MotionSts)  "<MotionSts>"
  Zero1/1 -> Assignment1/1
  Constant/1 -> Assignment1/3
  Assignment1/1 -> ACC_PO/1
  PO_K1/1 -> Selector1/1
  Constant1/1 -> Selector1/2
  Selector1/1 -> Bus Selector1/1

== system AccTarSel_PLAN_CTRL/calcCancelFlag ==
  MainState : Inport
  SYS_Info : Inport  Port=2
  AND : Logic  AllPortsSameDT=off  OutDataTypeStr=boolean
  Constant : Constant  Value=2  OutDataTypeStr=single
  Constant1 : Constant  OutDataTypeStr=single
  Constant2 : Constant  Value=0  OutDataTypeStr=single
  If : If  NumInputs=2  IfExpression=u1 ==1  ElseIfExpressions=u2 == 1
  If Action Subsystem : Subsystem  TreatAsAtomicUnit=on
  If Action Subsystem1 : Subsystem  TreatAsAtomicUnit=on
  If Action Subsystem2 : Subsystem  TreatAsAtomicUnit=on
  Memory : Memory
  Memory1 : Memory
  Merge : Merge  Inputs=3
  Merge1 : Merge  Inputs=3
  Relational Operator : RelationalOperator  OutDataTypeStr=boolean  RndMeth=Simplest
  Relational Operator1 : RelationalOperator  Operator=<=  OutDataTypeStr=boolean  RndMeth=Simplest
  Relational Operator2 : RelationalOperator  Operator=>  OutDataTypeStr=boolean  RndMeth=Simplest
  Cancel : Outport
  wires:
  MainState/1 -> Relational Operator1/1, Memory/1
  Constant/1 -> Relational Operator/2
  Memory/1 -> Relational Operator/1
  Constant1/1 -> Relational Operator1/2
  Relational Operator/1 -> AND/1
  Relational Operator1/1 -> AND/2
  AND/1 -> If/1
  If/1 -> If Action Subsystem/Action
  If Action Subsystem/1(CancelFlag) -> Merge/1
  If Action Subsystem1/1(CancelFlag) -> Merge/2
  If Action Subsystem2/1(CancelFlag) -> Merge/3
  If Action Subsystem/2(HoldTime) -> Merge1/1
  If Action Subsystem1/2(HoldTime) -> Merge1/2
  If Action Subsystem2/2(HoldTime) -> Merge1/3
  Merge1/1 -> Memory1/1
  SYS_Info/1 -> If Action Subsystem1/1(SYS_Info)
  Memory1/1 -> Relational Operator2/1, If Action Subsystem1/2(HoldTimeK1)
  If/2 -> If Action Subsystem1/Action
  If/3 -> If Action Subsystem2/Action
  Merge/1 -> Cancel/1
  Constant2/1 -> Relational Operator2/2
  Relational Operator2/1 -> If/2

== system AccTarSel_PLAN_CTRL/ACC_Target_Selection/Subsystem ==
  objInfo : Inport
  egoTrajLane_st : Inport  Port=2
  VSI_VehState_st : Inport  Port=3
  ATS_Internal_K1 : Inport  Port=4
  SYS_Info_st : Inport  Port=5
  ValidObjCalc : Subsystem  TreatAsAtomicUnit=on
  isTargetValid : Outport
  "ats_objInfo " : Outport  Port=2
  wires:
  ValidObjCalc/2("ats_objInfo ") -> "ats_objInfo "/1
  objInfo/1 -> ValidObjCalc/1(objInfo)
  egoTrajLane_st/1 -> ValidObjCalc/2(In2)
  ValidObjCalc/1(isTargetValid) -> isTargetValid/1
  VSI_VehState_st/1 -> ValidObjCalc/3(In3)
  ATS_Internal_K1/1 -> ValidObjCalc/4(ATS_Internal_K1)
  SYS_Info_st/1 -> ValidObjCalc/5(SYS_Info_st)

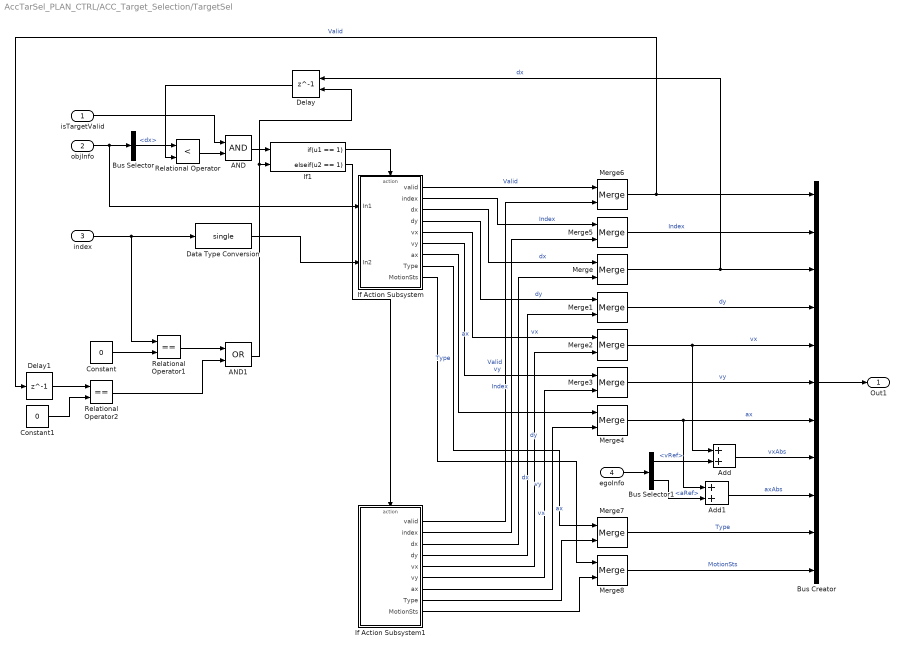
== system AccTarSel_PLAN_CTRL/ACC_Target_Selection/TargetSel ==
  isTargetValid : Inport
  objInfo : Inport  Port=2
  index : Inport  Port=3
  egoInfo : Inport  Port=4
  AND : Logic  AllPortsSameDT=off  OutDataTypeStr=boolean
  AND1 : Logic  Operator=OR  AllPortsSameDT=off  OutDataTypeStr=boolean
  Add : Sum
  Add1 : Sum
  Bus Creator : BusCreator  Inputs=11  OutDataTypeStr=Bus: ATS_PO_ST  NonVirtualBus=on
      settings: InheritFromInputs=off
  Bus Selector : BusSelector  OutputSignals=dx
  Bus Selector1 : BusSelector  OutputSignals=vRef,aRef
  Constant : Constant  Value=0  OutDataTypeStr=int32
  Constant1 : Constant  Value=0  OutDataTypeStr=boolean
  Data Type Conversion : DataTypeConversion  OutDataTypeStr=single
  Delay : Delay  DelayLength=1  InitialCondition=65535  ExternalReset=Level hold
      settings: InputPortMap=u0,r5
  Delay1 : Delay  DelayLength=1  InitialCondition=0
  If Action Subsystem : Subsystem  TreatAsAtomicUnit=on
  If Action Subsystem1 : Subsystem  TreatAsAtomicUnit=on
  If1 : If  NumInputs=2  IfExpression=u1 == 1  ElseIfExpressions=u2 == 1  ShowElse=off
  Merge{,1..8} (9 alike) : Merge
  Relational Operator : RelationalOperator  Operator=<  OutDataTypeStr=boolean  RndMeth=Simplest
  Relational Operator1 : RelationalOperator  Operator===  OutDataTypeStr=boolean  RndMeth=Simplest
  Relational Operator2 : RelationalOperator  Operator===  OutDataTypeStr=boolean  RndMeth=Simplest
  Out1 : Outport  OutDataTypeStr=Bus: ATS_PO_ST
  wires:
  isTargetValid/1 -> AND/1
  objInfo/1 -> If Action Subsystem/1(In1), Bus Selector/1
  Bus Selector/1 -> Relational Operator/1  "<dx>"
  index/1 -> Relational Operator1/1, Data Type Conversion/1
  If1/1 -> If Action Subsystem/Action
  Delay/1 -> Relational Operator/2
  Relational Operator/1 -> AND/2
  AND/1 -> If1/1
  Bus Creator/1 -> Out1/1
  Data Type Conversion/1 -> If Action Subsystem/2(In2)
  Constant/1 -> Relational Operator1/2
  AND1/1 -> Delay/2, If1/2
  If1/2 -> If Action Subsystem1/Action
  If Action Subsystem/3(dx) -> Merge/1  "dx"
  If Action Subsystem/4(dy) -> Merge1/1  "dy"
  If Action Subsystem/5(vx) -> Merge2/1  "vx"
  If Action Subsystem/6(vy) -> Merge3/1  "vy"
  If Action Subsystem/7(ax) -> Merge4/1  "ax"
  If Action Subsystem/2(index) -> Merge5/1  "Index"
  If Action Subsystem/1(valid) -> Merge6/1  "Valid"
  Merge6/1 -> Delay1/1, Bus Creator/1  "Valid"
  Merge5/1 -> Bus Creator/2  "Index"
  Merge/1 -> Delay/1, Bus Creator/3  "dx"
  Merge1/1 -> Bus Creator/4  "dy"
  Merge2/1 -> Add/1, Bus Creator/5  "vx"
  Merge3/1 -> Bus Creator/6  "vy"
  Merge4/1 -> Add1/1, Bus Creator/7  "ax"
  If Action Subsystem1/1(valid) -> Merge6/2  "Valid"
  If Action Subsystem1/2(index) -> Merge5/2  "Index"
  If Action Subsystem1/3(dx) -> Merge/2  "dx"
  If Action Subsystem1/4(dy) -> Merge1/2  "dy"
  If Action Subsystem1/5(vx) -> Merge2/2  "vx"
  If Action Subsystem1/6(vy) -> Merge3/2  "vy"
  If Action Subsystem1/7(ax) -> Merge4/2  "ax"
  If Action Subsystem1/8(Type) -> Merge7/2
  If Action Subsystem/8(Type) -> Merge7/1  "Type"
  Merge7/1 -> Bus Creator/10  "Type"
  Relational Operator1/1 -> AND1/1
  Constant1/1 -> Relational Operator2/2
  Delay1/1 -> Relational Operator2/1
  Relational Operator2/1 -> AND1/2
  egoInfo/1 -> Bus Selector1/1
  Bus Selector1/1 -> Add/2  "<vRef>"
  Add/1 -> Bus Creator/8  "vxAbs"
  Add1/1 -> Bus Creator/9  "axAbs"
  Bus Selector1/2 -> Add1/2  "<aRef>"
  If Action Subsystem/9(MotionSts) -> Merge8/1
  If Action Subsystem1/9(MotionSts) -> Merge8/2
  Merge8/1 -> Bus Creator/11  "MotionSts"

== system AccTarSel_PLAN_CTRL/ACC_dTarSet1/If Action Subsystem ==
  In1 : Inport
  Action Port : ActionPort  ActionType=then
  Add : Sum
  Constant : Constant  OutDataTypeStr=single
  Constant1 : Constant  Value=3  OutDataTypeStr=single
  Max : MinMax  Inputs=2
  Out1 : Outport
  wires:
  In1/1 -> Add/1
  Constant/1 -> Add/2
  Max/1 -> Out1/1
  Add/1 -> Max/1
  Constant1/1 -> Max/2

== system AccTarSel_PLAN_CTRL/ACC_dTarSet1/If Action Subsystem1 ==
  In1 : Inport
  Action Port : ActionPort  ActionType=elseif
  Add : Sum  Inputs=+-
  Constant : Constant  OutDataTypeStr=single
  Constant1 : Constant  OutDataTypeStr=single
  Max : MinMax  Function=max  Inputs=2
  Out1 : Outport
  wires:
  In1/1 -> Add/1
  Constant/1 -> Add/2
  Add/1 -> Max/1
  Max/1 -> Out1/1
  Constant1/1 -> Max/2

== system AccTarSel_PLAN_CTRL/ACC_dTarSet1/If Action Subsystem2 ==
  In1 : Inport
  Action Port : ActionPort  ActionType=else
  Out1 : Outport
  wires:
  In1/1 -> Out1/1

== system AccTarSel_PLAN_CTRL/ACC_dTarSet1/Subsystem ==
  ACCState : Inport
  Constant : Constant  Value=2  OutDataTypeStr=single
  Equal1 : RelationalOperator  Operator===  OutDataTypeStr=boolean  RndMeth=Simplest
  PreCon : Outport
  wires:
  Constant/1 -> Equal1/2
  ACCState/1 -> Equal1/1
  Equal1/1 -> PreCon/1

== system AccTarSel_PLAN_CTRL/Choose Exponential/Exponential ==
  EgoMotion : Inport
  ACC_STM : Inport  Port=2
  SYS_Info : Inport  Port=3
  Bus Selector : BusSelector  OutputSignals=vSet
  Subsystem : Subsystem
  Subsystem1 : Subsystem
  aCmd : Outport
  wires:
  ACC_STM/1 -> Bus Selector/1
  Bus Selector/1 -> [vSet], Subsystem/1(<vSet>)  "<vSet>"
  EgoMotion/1 -> [EgoMotion], Subsystem/2(EgoMotion)
  Subsystem/2(T1) -> Subsystem1/2(T1)
  Subsystem/1(T0) -> Subsystem1/1(T0)
  Subsystem/3(T2) -> Subsystem1/3(T2)
  SYS_Info/1 -> Subsystem1/4(SYS_Info)
  [vSet] -> Subsystem1/5(vSet)
  [EgoMotion] -> Subsystem1/6(EgoMotion)
  Subsystem1/1(aCmd) -> aCmd/1

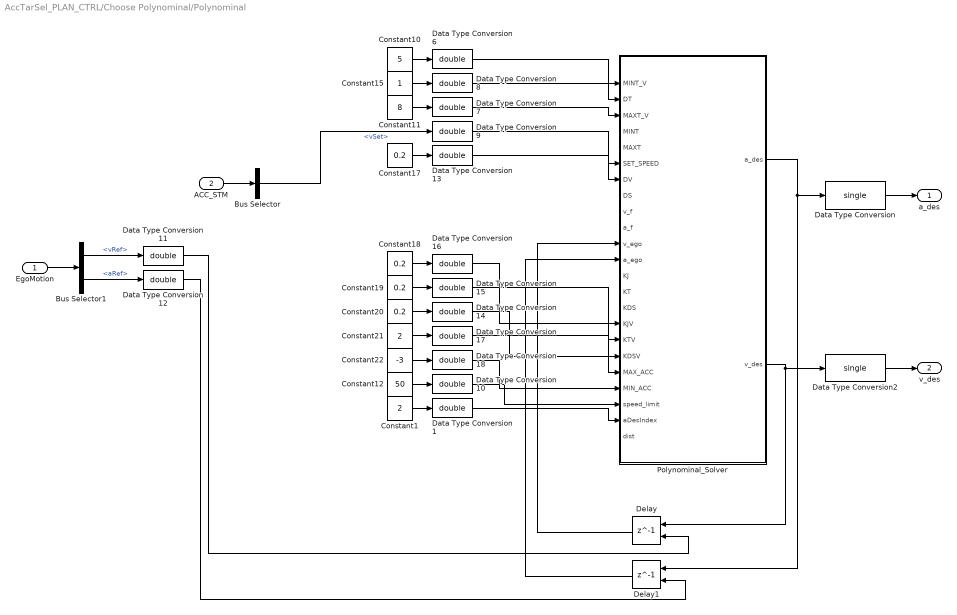
== system AccTarSel_PLAN_CTRL/Choose Polynominal/Polynominal ==
  EgoMotion : Inport
  ACC_STM : Inport  Port=2
  Bus Selector : BusSelector  OutputSignals=vSet
  Bus Selector1 : BusSelector  OutputSignals=vRef,aRef
  Constant1 : Constant  Value=2  OutDataTypeStr=single
  Constant10 : Constant  Value=5  OutDataTypeStr=single
  Constant11 : Constant  Value=8  OutDataTypeStr=single
  Constant12 : Constant  Value=50  OutDataTypeStr=single
  Constant15 : Constant  OutDataTypeStr=single
  Constant{17..20} (4 alike) : Constant  Value=0.2  OutDataTypeStr=single
  Constant21 : Constant  Value=2  OutDataTypeStr=single
  Constant22 : Constant  Value=-3  OutDataTypeStr=single
  Data Type Conversion : DataTypeConversion  OutDataTypeStr=single
  Data Type Conversion{1,6..18} (14 alike) : DataTypeConversion  OutDataTypeStr=double
  Data Type Conversion2 : DataTypeConversion  OutDataTypeStr=single
  Delay : Delay  DelayLength=1  InitialConditionSource=Input port
      settings: InputPortMap=u0,p4
  Delay1 : Delay  DelayLength=1  InitialConditionSource=Input port
      settings: InputPortMap=u0,p4
  Polynominal_Solver : MATLAB Function  TreatAsAtomicUnit=on
  a_des : Outport
  v_des : Outport  Port=2
  wires:
  Bus Selector/1 -> Data Type Conversion9/1  "<vSet>"
  Constant12/1 -> Data Type Conversion10/1
  Constant22/1 -> Data Type Conversion18/1
  Constant19/1 -> Data Type Conversion15/1
  Data Type Conversion17/1 -> Polynominal_Solver/19(MAX_ACC)
  Data Type Conversion14/1 -> Polynominal_Solver/18(KDSV)
  Data Type Conversion10/1 -> Polynominal_Solver/21(speed_limit)
  Data Type Conversion18/1 -> Polynominal_Solver/20(MIN_ACC)
  Constant17/1 -> Data Type Conversion13/1
  Constant20/1 -> Data Type Conversion14/1
  Data Type Conversion7/1 -> Polynominal_Solver/3(MAXT_V)
  Data Type Conversion11/1 -> Delay/2
  Constant21/1 -> Data Type Conversion17/1
  Bus Selector1/2 -> Data Type Conversion12/1  "<aRef>"
  Data Type Conversion6/1 -> Polynominal_Solver/1(MINT_V)
  Data Type Conversion15/1 -> Polynominal_Solver/17(KTV)
  Constant15/1 -> Data Type Conversion8/1
  Constant18/1 -> Data Type Conversion16/1
  Constant11/1 -> Data Type Conversion7/1
  Data Type Conversion9/1 -> Polynominal_Solver/6(SET_SPEED)
  Constant10/1 -> Data Type Conversion6/1
  Data Type Conversion13/1 -> Polynominal_Solver/7(DV)
  Data Type Conversion8/1 -> Polynominal_Solver/2(DT)
  Data Type Conversion16/1 -> Polynominal_Solver/16(KJV)
  Data Type Conversion12/1 -> Delay1/2
  Polynominal_Solver/1(a_des) -> Data Type Conversion/1, Delay1/1
  ACC_STM/1 -> Bus Selector/1
  EgoMotion/1 -> Bus Selector1/1
  Bus Selector1/1 -> Data Type Conversion11/1  "<vRef>"
  Data Type Conversion/1 -> a_des/1
  Constant1/1 -> Data Type Conversion1/1
  Data Type Conversion1/1 -> Polynominal_Solver/22(aDesIndex)
  Delay/1 -> Polynominal_Solver/11(v_ego)
  Data Type Conversion2/1 -> v_des/1
  Polynominal_Solver/2(v_des) -> Delay/1, Data Type Conversion2/1
  Delay1/1 -> Polynominal_Solver/12(a_ego)
  ? -> Polynominal_Solver/23(dist)
